simulink library "TemperatureLabLibrary"  (R2018b)
settings: Solver=VariableStepAuto  StartTime=0.0  StopTime=10.0  RelTol=1e-3
libraries: realtime_pacer_lib x1
settings Model: Creator=jarico  LastModifiedBy=jarico

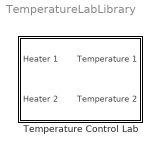
== system TemperatureLabLibrary ==
  Temperature Control Lab : Subsystem  mask(SISTEMA DE CONTROL DE TEMPERATURA){maxQ1=100, maxQ2=100, maxT1=80, maxT2=80, uLED=40}
      mask prompts: maxQ1 "Potencia máxima Q1 (%)"; maxQ2 "Potencia máxima Q2 (%)"; maxT1 "Temperatura máxima T1 (ºC)"; maxT2 "Temperatura máxima T2 (ºC)"; uLED "Temperatura umbral para los indicadores luminosos (ºC)"
      mask help:
      | Ajuste la configuración del dispositivo en función de sus necesidades.
      | Por seguridad, se recomienda limitar la temperatura en los transistores a un valor máximo de 80ºC.

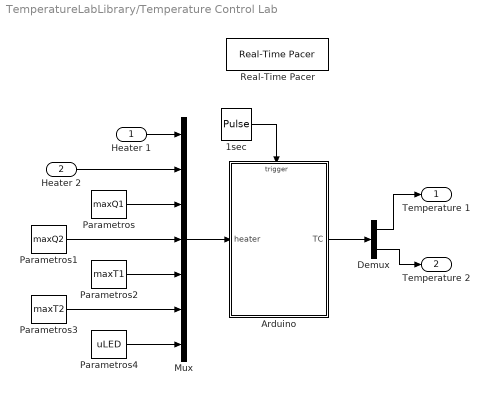
== system TemperatureLabLibrary/Temperature Control Lab ==
  Heater 1 : Inport
  Heater 2 : Inport  Port=2
  1sec : DiscretePulseGenerator  PulseType=Time based  Period=1  PulseWidth=50
  Arduino : Subsystem  TreatAsAtomicUnit=on
  Demux : Demux  Outputs=2
  Mux : Mux  Inputs=7
  Parametros : Constant  Value=maxQ1
  Parametros1 : Constant  Value=maxQ2
  Parametros2 : Constant  Value=maxT1
  Parametros3 : Constant  Value=maxT2
  Parametros4 : Constant  Value=uLED
  Real-Time Pacer : realtime_pacer_lib/Real-Time Pacer  simTimePerRealTime=1
  Temperature 1 : Outport
  Temperature 2 : Outport  Port=2
  wires:
  1sec/1 -> Arduino/Trigger
  Arduino/1(TC) -> Demux/1
  Heater 1/1 -> Mux/1
  Heater 2/1 -> Mux/2
  Mux/1 -> Arduino/1(heater)
  Demux/1 -> Temperature 1/1
  Demux/2 -> Temperature 2/1
  Parametros4/1 -> Mux/7
  Parametros3/1 -> Mux/6
  Parametros2/1 -> Mux/5
  Parametros1/1 -> Mux/4
  Parametros/1 -> Mux/3

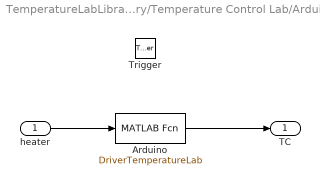
== system TemperatureLabLibrary/Temperature Control Lab/Arduino ==
  heater : Inport  LatchByDelayingOutsideSignal=on
  Trigger : TriggerPort  VariantControl=Variant
  Arduino : MATLABFcn  MATLABFcn=DriverTemperatureLab  OutputDimensions=2
  TC : Outport  InitialOutput=23
  wires:
  heater/1 -> Arduino/1
  Arduino/1 -> TC/1
